simulink model "EVmodel"  (R2022a)
settings: Solver=VariableStepAuto  StartTime=0.0  StopTime=1200  RelTol=1e-3  EnableMultiTasking=on
values from neighbouring files (symbols this model uses):
  eff_trans = 0.90    (= 0.9)    [Initial.m]
  Ki = 0.0    (= 0)    [Initial.m]
  Kp = 0.3    [Initial.m]
  r_gear = 9.34    [Initial.m]
undefined symbols (not defined in the file or in its folder): sigbuilder_block
libraries: simulink x2
settings Model: Creator=sunbignhan  LastModifiedBy=anthelion
settings SolverCC: AlgebraicLoopSolver=TrustRegion
settings DataIOCC: LimitDataPoints=on  SaveFormat=Array  SignalLoggingSaveFormat=ModelDataLogs  ReturnWorkspaceOutputs=off
settings OptimizationCC: InitFltsAndDblsToZero=on  LifeSpan=inf
settings DebuggingCC: SaveWithParameterizedLinksMsg=none  UnderspecifiedInitializationDetection=Classic  MergeDetectMultiDrivingBlocksExec=none  SignalResolutionControl=TryResolveAllWithWarning  MultiTaskDSMMsg=warning  MultiTaskCondExecSysMsg=none  FcnCallInpInsideContextMsg=warning  UnconnectedInputMsg=warning  UnconnectedOutputMsg=warning  UnconnectedLineMsg=warning  SFUnexpectedBacktrackingDiag=warning  SFNoUnconditionalDefaultTransitionDiag=warning  SFExecutionAtInitializationDiag=none  SFMachineParentedDataDiag=warning  ArithmeticOperatorsInVariantConditions=warning
settings HardwareCC: ProdBitPerPointer=32  ProdBitPerSizeT=32  ProdBitPerPtrDiffT=32  ProdLargestAtomicFloat=None  ProdIntDivRoundTo=Undefined  ProdEndianess=Unspecified  ProdWordSize=32  ProdHWDeviceType=32-bit Generic
settings ModelReferenceCC: PropagateSignalLabelsOutOfModel=off
settings RTWCC: DLArmComputeVersion=19.05
settings CodeAppCC: StateflowObjectComments=on
settings GRTTargetCC: TargetFcnLib=ansi_tfl_tmw.mat  TargetLangStandard=C89/C90 (ANSI)  CombineOutputUpdateFcns=off  GRTInterface=on
settings ConfigComp: CovMetricSettings=dw  CovSaveCumulativeToWorkspaceVar=on  CovSaveSingleToWorkspaceVar=on

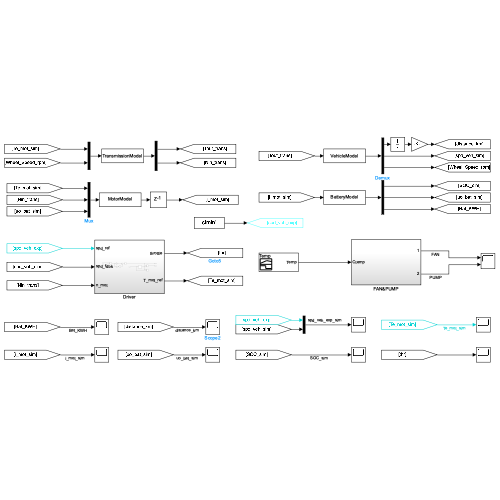
[thumbnail: Simulink's stored preview of the top-level diagram]
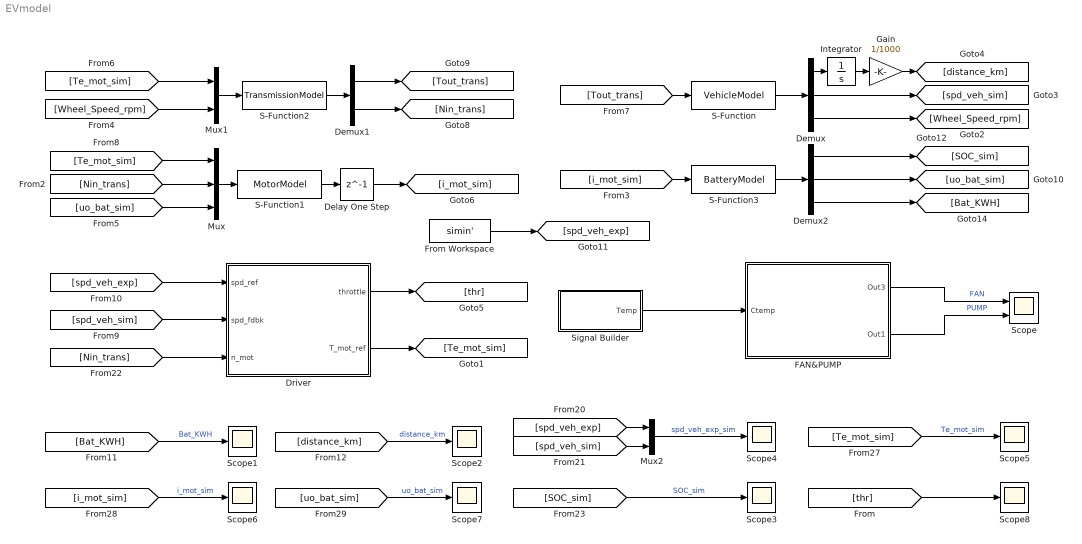
== system EVmodel ==
  Delay One Step : Delay  DelayLength=1
  Demux : Demux  Outputs=3
  Demux1 : Demux  Outputs=2
  Demux2 : Demux  Outputs=3
  Driver : Subsystem
  FAN&PUMP : Subsystem
  From Workspace : FromWorkspace  VariableName=simin'
  Gain : Gain  Gain=1/1000
  Integrator : Integrator
  Mux : Mux  Inputs=3
  Mux1 : Mux  Inputs=2
  Mux2 : Mux  Inputs=2
  S-Function : S-Function  FunctionName=VehicleModel  Parameters=r_Wheel, A_Drag,f0,g,m  SFunctionDeploymentMode=off  EnableBusSupport=off
  S-Function1 : S-Function  FunctionName=MotorModel  SFunctionDeploymentMode=off  EnableBusSupport=off
  S-Function2 : S-Function  FunctionName=TransmissionModel  Parameters=r_gear,eff_trans  SFunctionDeploymentMode=off  EnableBusSupport=off
  S-Function3 : S-Function  FunctionName=BatteryModel  Parameters=SOC_initial, Bat_Cap_Ah  SFunctionDeploymentMode=off  EnableBusSupport=off
  Scope : Scope  NumInputPorts=2
  Scope{1..8} (8 alike) : Scope
  Signal Builder : Subsystem  Tag=STV Subsys  LoadFcn=sigbuilder_block('load');  StartFcn=sigbuilder_block('start');  StopFcn=sigbuilder_block('stop');  ClipboardFcn=sigbuilder_block('clipboard');  mask(Sigbuilder block){tuvar=[0:10]}
      mask help: Simulink:masks:SigbuilderBlock_MD
      mask init:
      | if ~strcmp(get_param(bdroot(gcbh),'SimulationStatus'),'stopped') tuvar = sigbuilder_block('maskInit'); end
      settings: CopyFcn=sigbuilder_block('copy');  DeleteFcn=sigbuilder_block('delete');  ModelCloseFcn=sigbuilder_block('modelClose');  PreSaveFcn=sigbuilder_block('preSave');  PauseFcn=sigbuilder_block('pause');  ContinueFcn=sigbuilder_block('continue');  NameChangeFcn=sigbuilder_block('namechange');  OpenFcn=sigbuilder_block('open',[231 121 949 345 ]);  CloseFcn=sigbuilder_block('close');
      mask Display: plot(0, 0, 100, 100,[2, 2, 32, 32, 2], [68, 8, 8, 68, 68],[32, 2], [38, 38], [32, 19, 2],[53, 60, 44], [32, 17, 17, 2],[16, 16, 31, 31]);txt = getActiveGroup(gcbh);text(2, 100, txt,'verticalAlignment', 'top');
  wires:
  From Workspace/1 -> [spd_veh_exp]
  [Bat_KWH] -> Scope1/1  "Bat_KWH"
  [distance_km] -> Scope2/1  "distance_km"
  [SOC_sim] -> Scope3/1  "SOC_sim"
  [spd_veh_sim] -> Mux2/2
  [spd_veh_exp] -> Mux2/1
  Mux2/1 -> Scope4/1  "spd_veh_exp_sim"
  [Te_mot_sim] -> Scope5/1  "Te_mot_sim"
  [i_mot_sim] -> Scope6/1  "i_mot_sim"
  [uo_bat_sim] -> Scope7/1  "uo_bat_sim"
  Signal Builder/1(Temp) -> FAN&PUMP/1(Ctemp)
  FAN&PUMP/1(Out3) -> Scope/1  "FAN"
  FAN&PUMP/2(Out1) -> Scope/2  "PUMP"
  [Tout_trans] -> S-Function/1
  S-Function/1 -> Demux/1
  Demux/1 -> Integrator/1
  Integrator/1 -> Gain/1
  Demux/3 -> [Wheel_Speed_rpm]
  Gain/1 -> [distance_km]
  [Nin_trans] -> Mux/2
  [Te_mot_sim] -> Mux/1
  [uo_bat_sim] -> Mux/3
  Mux/1 -> S-Function1/1
  S-Function1/1 -> Delay One Step/1
  Mux1/1 -> S-Function2/1
  [Te_mot_sim] -> Mux1/1
  [Wheel_Speed_rpm] -> Mux1/2
  S-Function2/1 -> Demux1/1
  Demux1/1 -> [Tout_trans]
  [i_mot_sim] -> S-Function3/1
  S-Function3/1 -> Demux2/1
  Demux2/1 -> [SOC_sim]
  Demux2/2 -> [uo_bat_sim]
  Demux2/3 -> [Bat_KWH]
  Delay One Step/1 -> [i_mot_sim]
  Demux1/2 -> [Nin_trans]
  Demux/2 -> [spd_veh_sim]
  [spd_veh_exp] -> Driver/1(spd_ref)
  [spd_veh_sim] -> Driver/2(spd_fdbk)
  [Nin_trans] -> Driver/3(n_mot)
  Driver/1(throttle) -> [thr]
  Driver/2(T_mot_ref) -> [Te_mot_sim]
  [thr] -> Scope8/1

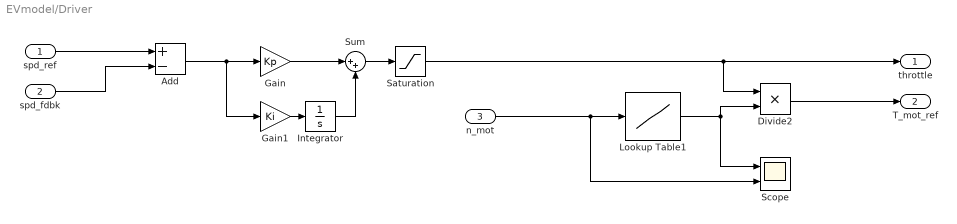
== system EVmodel/Driver ==
  spd_ref : Inport
  spd_fdbk : Inport  Port=2
  n_mot : Inport  Port=3
  Add : Sum  Inputs=+-
  Divide2 : Product  Inputs=**
  Gain : Gain  Gain=Kp
  Gain1 : Gain  Gain=Ki
  Integrator : Integrator
  Lookup Table1 : Lookup  InputValues=[517 1021 2009 3247 4024 5025 6023 7017 8021 9008 10027]  Table=[173.1 172 170.5 168.4 137.1 111.4 97.4 84.3 72.7 63.8 57.8]  SaturateOnIntegerOverflow=off
  Saturation : Saturate  UpperLimit=1  LowerLimit=-1
  Scope : Scope  NumInputPorts=2
  Sum : Sum  Inputs=|++
  throttle : Outport
  T_mot_ref : Outport  Port=2
  wires:
  spd_ref/1 -> Add/1
  spd_fdbk/1 -> Add/2
  Integrator/1 -> Sum/2
  Gain1/1 -> Integrator/1
  Sum/1 -> Saturation/1
  Gain/1 -> Sum/1
  Add/1 -> Gain1/1, Gain/1
  Saturation/1 -> Divide2/1, throttle/1
  n_mot/1 -> Scope/2, Lookup Table1/1
  Lookup Table1/1 -> Scope/1, Divide2/2
  Divide2/1 -> T_mot_ref/1

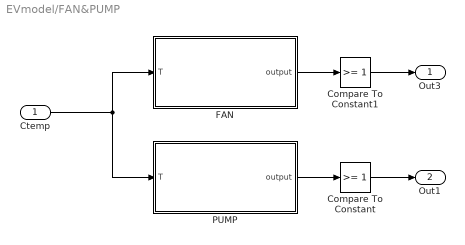
== system EVmodel/FAN&PUMP ==
  Ctemp : Inport
  Compare To Constant : simulink/Logic and Bit Operations/Compare To Constant  relop=>=  const=1  OutDataTypeStr=boolean
  Compare To Constant1 : simulink/Logic and Bit Operations/Compare To Constant  relop=>=  const=1  OutDataTypeStr=boolean
  FAN : Stateflow chart  TreatAsAtomicUnit=on
  PUMP : Stateflow chart  TreatAsAtomicUnit=on
  Out3 : Outport
  Out1 : Outport  Port=2
  wires:
  Ctemp/1 -> FAN/1(T), PUMP/1(T)
  FAN/1(output) -> Compare To Constant1/1
  Compare To Constant1/1 -> Out3/1
  Compare To Constant/1 -> Out1/1
  PUMP/1(output) -> Compare To Constant/1

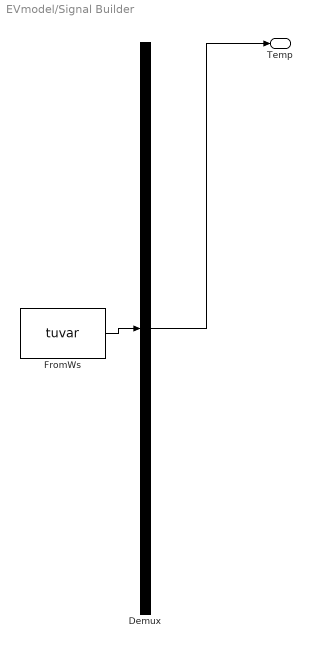
== system EVmodel/Signal Builder ==
  Demux : Demux  Tag=STV Demux  Outputs=1
      settings: DisplayOption=none
  FromWs : FromWorkspace  Tag=STV FromWs  VariableName=tuvar
      SigBuilderData=|
      | common.afterFinalStr = 'Extrapolate'
      | common.sampleTime = 0
      | dataSet.timeRange = [0 1200]
      | dataSet.name = 'Temp'
      | sbobj.Groups.Name = 'Temp'
      | sbobj.Groups.Signals.Name = 'Temp'
      | sbobj.Groups.Signals.XData = [0 200 400 600 700 900 1000 1200]
      | sbobj.Groups.Signals.YData = [0 45 80 38.5 60 10 5.5 0]
      | sbobj.Groups.TimeRange = [0 1200]
  Temp : Outport  Tag=STV Outport
  wires:
  Demux/1 -> Temp/1
  FromWs/1 -> Demux/1

== stateflow chart EVmodel/FAN&PUMP/PUMP ==
  state PUMP_STOP
    output=0;
  state PUMP_START
    output=1;
  (default) -> (junction 5) [commented out]
  (default) -> PUMP_STOP
  (junction 5) -> (junction 6) [commented out] : [T>=20]
  PUMP_STOP -> PUMP_START : [T>=20]
  (junction 5) -> (junction 7) [commented out] : [T<=10]
  (junction 6) -> (junction 8) [commented out] : {output=1;}
  PUMP_START -> PUMP_STOP : [T<=10]
  (junction 8) -> (junction 1) [commented out]
  (junction 7) -> (junction 1) [commented out] : {output=0;}
  data: output output; T input

== stateflow chart EVmodel/FAN&PUMP/FAN ==
  state FAN_STOP
    output=0;
  state FAN_START
    output=1;
  (default) -> FAN_STOP
  (default) -> (junction 5) [commented out]
  FAN_STOP -> FAN_START : [T>=55]
  (junction 5) -> (junction 6) [commented out] : [T>=55]
  (junction 5) -> (junction 7) [commented out] : [T<=45]
  (junction 6) -> (junction 8) [commented out] : {output=1;}
  FAN_START -> FAN_STOP : [T<=45]
  (junction 8) -> (junction 1) [commented out]
  (junction 7) -> (junction 1) [commented out] : {output=0;}
  data: output output; T input
